simulink model "sampleModel1979_5"  (R2023a)
settings: Solver=VariableStepAuto  StartTime=0.0  StopTime=10.0  RelTol=1e-3
libraries: hdlsllib x6, simulink x2
settings Model: Creator=user1  LastModifiedBy=user1

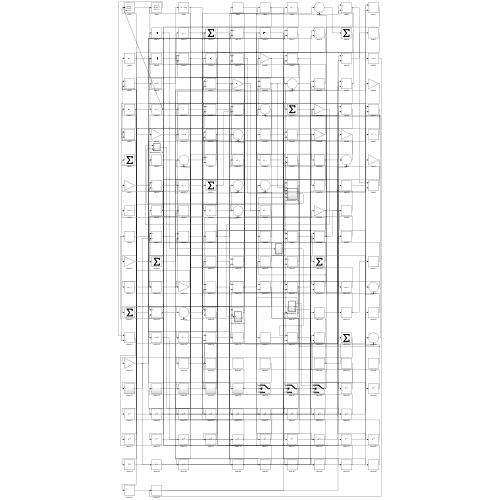
[thumbnail: Simulink's stored preview of the top-level diagram]
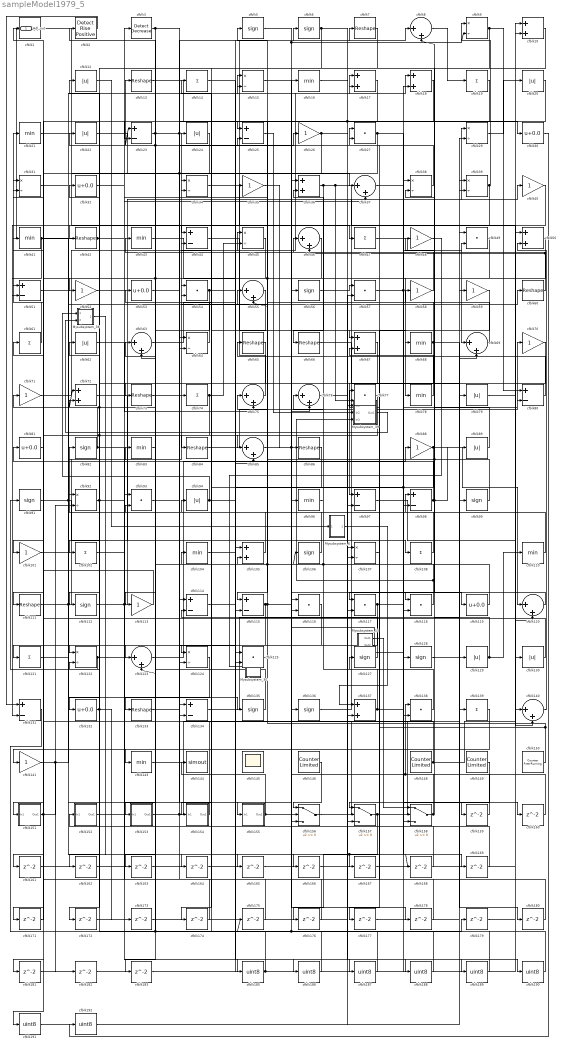
== system sampleModel1979_5 ==
  Mysubsystem_15 : Subsystem  TreatAsAtomicUnit=on  RTWFcnName=Mysubsystem_15
      settings: RTWFcnNameOpts=User specified  RTWFileNameOpts=Use function name
  Mysubsystem_30 : Subsystem  TreatAsAtomicUnit=on  RTWFcnName=Mysubsystem_30
      settings: RTWFcnNameOpts=User specified  RTWFileNameOpts=Use function name
  Mysubsystem_36 : Subsystem  TreatAsAtomicUnit=on  RTWFcnName=Mysubsystem_36
      settings: RTWFcnNameOpts=User specified  RTWFileNameOpts=Use function name
  Mysubsystem_39 : Subsystem  TreatAsAtomicUnit=on  RTWFcnName=Mysubsystem_39
      settings: RTWFcnNameOpts=User specified  RTWFileNameOpts=Use function name
  Mysubsystem_6 : Subsystem  TreatAsAtomicUnit=on  RTWFcnName=Mysubsystem_6
      settings: RTWFcnNameOpts=User specified  RTWFileNameOpts=Use function name
  cfblk1 : simulink/Logic and Bit Operations/Bit Set  iBit=0
      settings: LibrarySourceBlock=|
      | hdlsllib/Logic and Bit
      | Operations/Bit Set
  cfblk{10,17..18,36,50,67,72,105,137} (9 alike) : Sum  OutDataTypeStr=uint8
  cfblk{26,35,40,48,52,58..59,70..71,88,101,113,141} (13 alike) : Gain  OutDataTypeStr=uint8
  cfblk{14,19,47,61,74,102,108,121,139} (9 alike) : Sum  Inputs=+  OutDataTypeStr=uint8
  cfblk{16,21,41,43,68,78,83,96,104,110,143} (11 alike) : MinMax  OutDataTypeStr=uint8
  cfblk{5..6,56,82,91,99,106,112,127..128,135..136} (12 alike) : Signum
  cfblk{9,15,29,31,34,38..39,45,64,92,107,122,124} (13 alike) : Product  Inputs=*/  OutDataTypeStr=uint8  RndMeth=Zero  SaturateOnIntegerOverflow=on
  cfblk{7,13,42,60,65..66,73,84,86,111,133} (11 alike) : Reshape
  cfblk{23,25,44,51,80,97..98,114..115,131,134} (11 alike) : Sum  Inputs=+-  OutDataTypeStr=uint8
  cfblk{27,49,54,57,77,93,116..118,125,138} (11 alike) : DotProduct  OutDataTypeStr=uint8
  cfblk{30,32,53,81,119,132} (6 alike) : Bias  Bias=0.0  SaturateOnIntegerOverflow=off
  cfblk{12,20,22,24,62,79,89,94,129..130} (10 alike) : Abs  OutDataTypeStr=uint8  SaturateOnIntegerOverflow=off
  cfblk{8,37,46,55,63,69,75..76,85,120,123,140} (12 alike) : Sum  Inputs=|++  OutDataTypeStr=uint8
  cfblk144 : ToWorkspace  VariableName=simout  SaveFormat=Timeseries  SampleTime=-1
  cfblk145 : Scope
      settings: Floating=on
  cfblk146 : hdlsllib/Sources/Counter Limited  uplimit=7  tsamp=-1
  cfblk148 : hdlsllib/Sources/Counter Limited  uplimit=7  tsamp=-1
  cfblk149 : hdlsllib/Sources/Counter Limited  uplimit=7  tsamp=-1
  cfblk150 : hdlsllib/Sources/Counter Free-Running  NumBits=16  tsamp=-1
  cfblk151 : Subsystem
      settings: LibrarySourceBlock=|
      | hdlsllib/Ports &
      | Subsystems/Subsystem
  cfblk152 : Subsystem
      settings: LibrarySourceBlock=|
      | hdlsllib/Ports &
      | Subsystems/Subsystem
  cfblk153 : Subsystem
      settings: LibrarySourceBlock=|
      | hdlsllib/Ports &
      | Subsystems/Subsystem
  cfblk154 : Subsystem
      settings: LibrarySourceBlock=|
      | hdlsllib/Ports &
      | Subsystems/Subsystem
  cfblk155 : Subsystem
      settings: LibrarySourceBlock=|
      | hdlsllib/Ports &
      | Subsystems/Subsystem
  cfblk156 : Switch  OutDataTypeStr=uint8  SaturateOnIntegerOverflow=off  InputSameDT=off
  cfblk157 : Switch  OutDataTypeStr=uint8  SaturateOnIntegerOverflow=off  InputSameDT=off
  cfblk158 : Switch  OutDataTypeStr=uint8  SaturateOnIntegerOverflow=off  InputSameDT=off
  cfblk{159..169,171..183} (24 alike) : Delay  SampleTime=1
  cfblk{185..192} (8 alike) : DataTypeConversion  OutDataTypeStr=uint8  SaturateOnIntegerOverflow=off  RndMeth=Floor
  cfblk2 : hdlsllib/Logic and Bit Operations/Detect Rise Positive  vinit=0  OutDataTypeStr=uint8
  cfblk3 : simulink/Logic and Bit Operations/Detect Decrease  vinit=0.0  OutDataTypeStr=uint8
      settings: LibrarySourceBlock=|
      | hdlsllib/Logic and Bit
      | Operations/Detect
      | Decrease
  Hdl_out : Outport  OutDataTypeStr=uint8
  wires:
  cfblk35/1 -> cfblk86/1
  cfblk75/1 -> cfblk6/1
  cfblk115/1 -> cfblk55/2, cfblk76/2, cfblk121/1
  cfblk150/1 -> cfblk75/1, cfblk127/1
  cfblk38/1 -> cfblk13/1
  cfblk106/1 -> cfblk82/1
  cfblk136/1 -> cfblk29/1
  cfblk112/1 -> cfblk40/1, cfblk15/2
  cfblk94/1 -> Mysubsystem_36/1(In1), cfblk7/1
  cfblk58/1 -> cfblk43/1
  cfblk73/1 -> cfblk24/1
  cfblk61/1 -> cfblk21/1
  cfblk102/1 -> cfblk34/1
  cfblk40/1 -> cfblk42/1
  cfblk1/1 -> cfblk96/1
  cfblk3/1 -> cfblk143/1, cfblk125/2
  cfblk77/1 -> cfblk122/1, cfblk151/1(In1)
  cfblk99/1 -> cfblk54/1, cfblk58/1
  cfblk137/1 -> cfblk106/1, cfblk76/1, cfblk169/1
  cfblk47/1 -> cfblk69/1
  cfblk122/1 -> cfblk91/1, cfblk186/1
  cfblk24/1 -> cfblk113/1
  cfblk70/1 -> cfblk97/1
  cfblk120/1 -> cfblk117/1
  cfblk29/1 -> cfblk20/1
  cfblk107/1 -> cfblk77/1
  cfblk52/1 -> cfblk18/1
  cfblk53/1 -> cfblk45/1
  cfblk123/1 -> cfblk88/1
  cfblk54/1 -> cfblk98/2, cfblk163/1
  cfblk84/1 -> cfblk70/1
  cfblk45/1 -> cfblk141/1, cfblk183/1
  cfblk111/1 -> cfblk74/1, cfblk17/2
  cfblk69/1 -> cfblk34/2
  cfblk153/1(Out1) -> cfblk99/1, cfblk8/1
  cfblk158/1 -> cfblk138/1, cfblk67/2, cfblk98/1
  cfblk60/1 -> cfblk46/1, cfblk46/2
  cfblk49/1 -> cfblk78/1
  cfblk39/1 -> cfblk9/1, cfblk51/2
  cfblk74/1 -> cfblk134/2, cfblk45/2
  cfblk56/1 -> cfblk57/1
  cfblk105/1 -> cfblk92/1
  cfblk13/1 -> cfblk25/1
  cfblk19/1 -> cfblk84/1
  cfblk6/1 -> cfblk112/1, cfblk119/1
  cfblk86/1 -> cfblk154/1(In1)
  cfblk129/1 -> cfblk48/1, cfblk110/1
  cfblk27/1 -> cfblk64/2, cfblk160/1
  cfblk135/1 -> cfblk71/1
  cfblk143/1 -> cfblk38/1
  cfblk110/1 -> cfblk94/1
  cfblk156/1 -> cfblk39/1
  cfblk149/1 -> cfblk157/1
  cfblk71/1 -> cfblk16/1
  cfblk130/1 -> cfblk61/1
  cfblk7/1 -> cfblk102/1
  cfblk118/1 -> Mysubsystem_39/3(In3), cfblk63/1
  cfblk132/1 -> cfblk172/1, cfblk173/1
  cfblk141/1 -> cfblk60/1, cfblk182/1
  cfblk72/1 -> cfblk114/1
  cfblk42/1 -> cfblk47/1, Hdl_out/1
  cfblk18/1 -> cfblk111/1
  cfblk82/1 -> cfblk167/1, cfblk168/1, cfblk72/2
  cfblk32/1 -> cfblk3/1
  cfblk80/1 -> cfblk65/1
  cfblk121/1 -> cfblk83/1
  cfblk78/1 -> cfblk27/1
  cfblk66/1 -> cfblk129/1
  cfblk8/1 -> cfblk19/1
  cfblk34/1 -> cfblk137/2
  cfblk125/1 -> cfblk25/2
  cfblk98/1 -> cfblk89/1, cfblk8/2, cfblk81/1
  cfblk92/1 -> cfblk32/1, cfblk37/2
  cfblk138/1 -> cfblk114/2
  cfblk20/1 -> cfblk85/1
  cfblk68/1 -> cfblk73/1, cfblk22/1, cfblk180/1
  cfblk104/1 -> cfblk189/1
  cfblk46/1 -> cfblk115/1, cfblk181/1
  cfblk43/1 -> cfblk105/1
  cfblk23/1 -> cfblk30/1, cfblk37/1, cfblk123/2
  cfblk16/1 -> cfblk97/2
  cfblk2/1 -> cfblk131/1
  cfblk146/1 -> cfblk156/1
  cfblk155/1(Out1) -> cfblk144/1, cfblk178/1
  cfblk15/1 -> cfblk136/1
  cfblk14/1 -> cfblk187/1
  cfblk85/1 -> cfblk56/1, cfblk117/2
  cfblk62/1 -> cfblk75/2
  cfblk5/1 -> cfblk9/2, cfblk67/1
  cfblk127/1 -> cfblk105/2
  cfblk36/1 -> cfblk140/2, cfblk77/2, cfblk66/1
  cfblk117/1 -> cfblk80/2, cfblk161/1
  cfblk157/1 -> cfblk69/2, cfblk176/1
  cfblk37/1 -> cfblk138/2
  cfblk26/1 -> cfblk171/1, cfblk188/1
  cfblk89/1 -> cfblk38/2
  cfblk55/1 -> cfblk124/1
  cfblk64/1 -> cfblk53/1
  cfblk21/1 -> cfblk124/2, cfblk116/2
  cfblk17/1 -> Mysubsystem_39/1(In1), cfblk23/2
  cfblk67/1 -> cfblk132/1
  cfblk57/1 -> cfblk49/2, cfblk159/1
  cfblk154/1(Out1) -> cfblk31/1
  cfblk10/1 -> cfblk118/1
  cfblk133/1 -> cfblk156/2
  cfblk113/1 -> cfblk51/1
  cfblk134/1 -> cfblk79/1
  cfblk124/1 -> cfblk153/1(In1)
  cfblk9/1 -> cfblk44/1, cfblk80/1
  cfblk140/1 -> cfblk50/2
  cfblk83/1 -> cfblk133/1
  cfblk79/1 -> cfblk10/1
  cfblk44/1 -> cfblk68/1
  cfblk31/1 -> cfblk15/1
  cfblk119/1 -> cfblk2/1, cfblk23/1, cfblk5/1
  cfblk128/1 -> cfblk59/1
  cfblk116/1 -> cfblk123/1
  cfblk96/1 -> cfblk36/2
  cfblk151/1(Out1) -> cfblk41/1, cfblk92/2
  cfblk22/1 -> cfblk107/2
  cfblk41/1 -> cfblk155/1(In1), cfblk131/2
  cfblk108/1 -> cfblk55/1
  cfblk91/1 -> cfblk108/1, cfblk17/1
  cfblk88/1 -> cfblk158/2, cfblk174/1, cfblk120/1
  cfblk148/1 -> cfblk62/1, cfblk72/1, cfblk130/1
  cfblk50/1 -> cfblk52/1
  cfblk81/1 -> cfblk101/1
  cfblk97/1 -> cfblk120/2
  cfblk63/1 -> cfblk35/1
  cfblk51/1 -> cfblk135/1
  cfblk152/1(Out1) -> cfblk185/1
  cfblk93/1 -> cfblk26/1
  cfblk159/1 -> cfblk36/1
  cfblk160/1 -> cfblk49/1
  cfblk161/1 -> cfblk18/2
  cfblk65/1 -> cfblk162/1
  cfblk162/1 -> cfblk134/1
  cfblk163/1 -> cfblk29/2
  cfblk101/1 -> cfblk164/1
  cfblk164/1 -> cfblk54/2
  cfblk165/1 -> cfblk57/2
  cfblk114/1 -> cfblk166/1
  cfblk166/1 -> cfblk107/1
  cfblk167/1 -> cfblk50/1
  cfblk168/1 -> cfblk122/2
  cfblk169/1 -> cfblk44/2
  cfblk171/1 -> cfblk1/1
  cfblk172/1 -> cfblk157/2
  cfblk173/1 -> cfblk115/2
  cfblk174/1 -> cfblk64/1
  cfblk175/1 -> cfblk93/1
  cfblk176/1 -> cfblk63/2
  cfblk59/1 -> cfblk177/1
  cfblk177/1 -> cfblk39/2
  cfblk178/1 -> cfblk31/2
  cfblk131/1 -> cfblk179/1
  cfblk179/1 -> cfblk140/1
  cfblk180/1 -> cfblk27/2
  cfblk181/1 -> cfblk118/2
  cfblk182/1 -> cfblk85/2
  cfblk183/1 -> cfblk10/2
  cfblk185/1 -> cfblk125/1, cfblk128/1
  cfblk186/1 -> cfblk152/1(In1)
  cfblk187/1 -> cfblk175/1, cfblk116/1
  cfblk188/1 -> cfblk14/1
  cfblk189/1 -> cfblk93/2, cfblk12/1
  cfblk76/1 -> cfblk190/1
  cfblk190/1 -> cfblk104/1
  cfblk139/1 -> cfblk191/1
  cfblk191/1 -> cfblk157/3
  cfblk30/1 -> cfblk192/1
  cfblk192/1 -> cfblk139/1
  cfblk12/1 -> Mysubsystem_6/1(In1)
  Mysubsystem_6/1(Out1) -> cfblk137/1
  Mysubsystem_15/1(Out1) -> cfblk158/1
  Mysubsystem_15/2(Out2) -> cfblk156/3
  Mysubsystem_15/3(Out3) -> cfblk158/3
  cfblk48/1 -> Mysubsystem_30/1(U)
  Mysubsystem_36/1(Out1) -> cfblk165/1
  cfblk25/1 -> Mysubsystem_39/2(In2)
  Mysubsystem_39/1(Out1) -> Mysubsystem_36/2(In2)

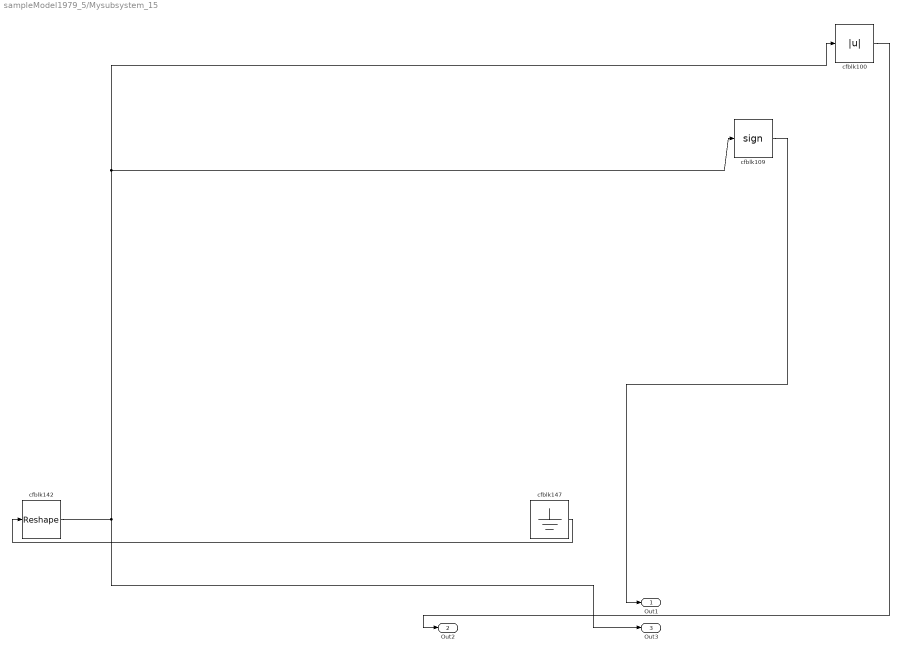
== system sampleModel1979_5/Mysubsystem_15 ==
  cfblk100 : Abs  SaturateOnIntegerOverflow=off
  cfblk109 : Signum
  cfblk142 : Reshape
  cfblk147 : Ground
  Out1 : Outport
  Out2 : Outport  Port=2
  Out3 : Outport  Port=3
  wires:
  cfblk109/1 -> Out1/1
  cfblk147/1 -> cfblk142/1
  cfblk142/1 -> Out3/1, cfblk109/1, cfblk100/1
  cfblk100/1 -> Out2/1

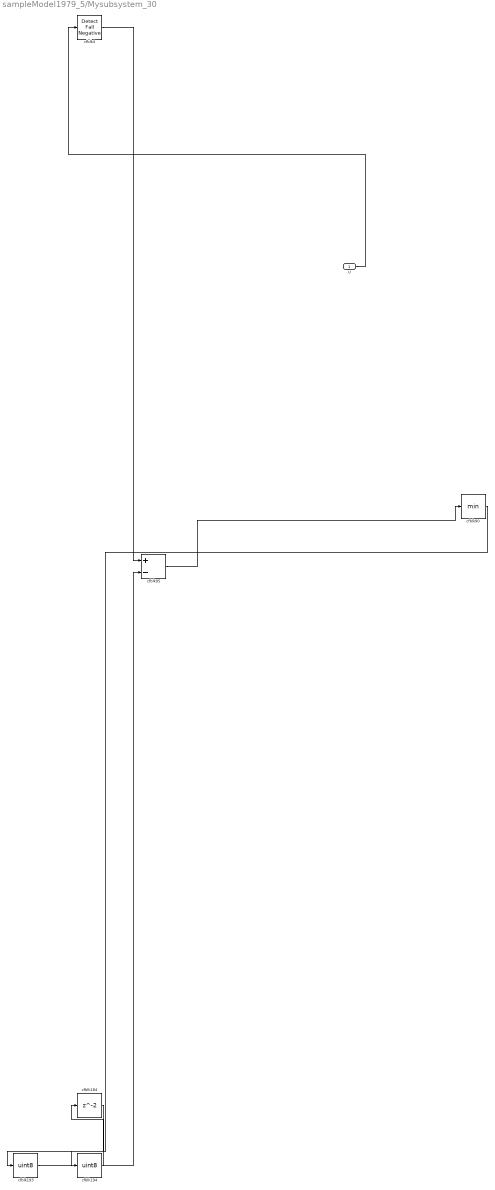
== system sampleModel1979_5/Mysubsystem_30 ==
  U : Inport
  cfblk184 : Delay  SampleTime=1
  cfblk193 : DataTypeConversion  OutDataTypeStr=uint8  SaturateOnIntegerOverflow=off  RndMeth=Floor
  cfblk194 : DataTypeConversion  OutDataTypeStr=uint8  SaturateOnIntegerOverflow=off  RndMeth=Floor
  cfblk4 : hdlsllib/Logic and Bit Operations/Detect Fall Negative  vinit=0  OutDataTypeStr=boolean
  cfblk90 : MinMax
  cfblk95 : Sum  Inputs=+-
  wires:
  cfblk184/1 -> cfblk193/1
  cfblk95/1 -> cfblk90/1
  cfblk4/1 -> cfblk95/1
  cfblk193/1 -> cfblk95/2
  cfblk194/1 -> cfblk184/1
  U/1 -> cfblk4/1
  cfblk90/1 -> cfblk194/1

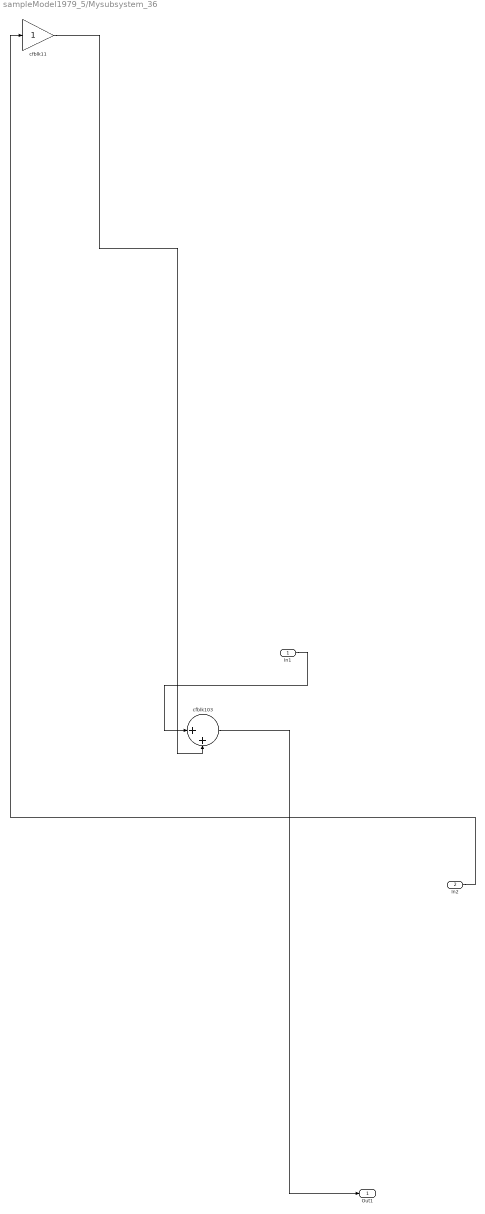
== system sampleModel1979_5/Mysubsystem_36 ==
  In1 : Inport
  In2 : Inport  Port=2
  cfblk103 : Sum  Inputs=|++
  cfblk11 : Gain
  Out1 : Outport
  wires:
  cfblk11/1 -> cfblk103/2
  In2/1 -> cfblk11/1
  In1/1 -> cfblk103/1
  cfblk103/1 -> Out1/1

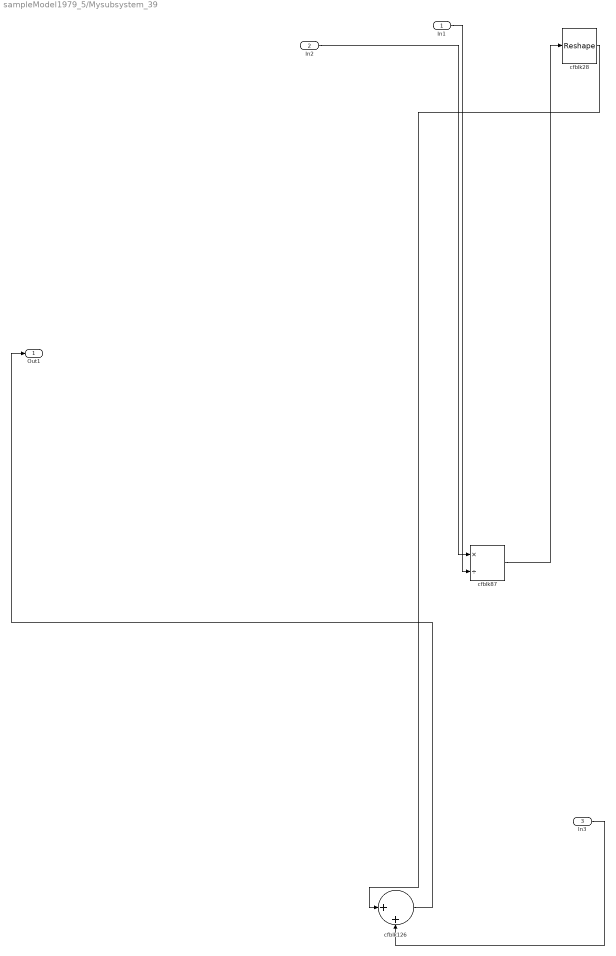
== system sampleModel1979_5/Mysubsystem_39 ==
  In1 : Inport
  In2 : Inport  Port=2
  In3 : Inport  Port=3
  cfblk126 : Sum  Inputs=|++
  cfblk28 : Reshape
  cfblk87 : Product  Inputs=*/  RndMeth=Zero  SaturateOnIntegerOverflow=on
  Out1 : Outport
  wires:
  cfblk28/1 -> cfblk126/1
  cfblk87/1 -> cfblk28/1
  In1/1 -> cfblk87/2
  cfblk126/1 -> Out1/1
  In3/1 -> cfblk126/2
  In2/1 -> cfblk87/1

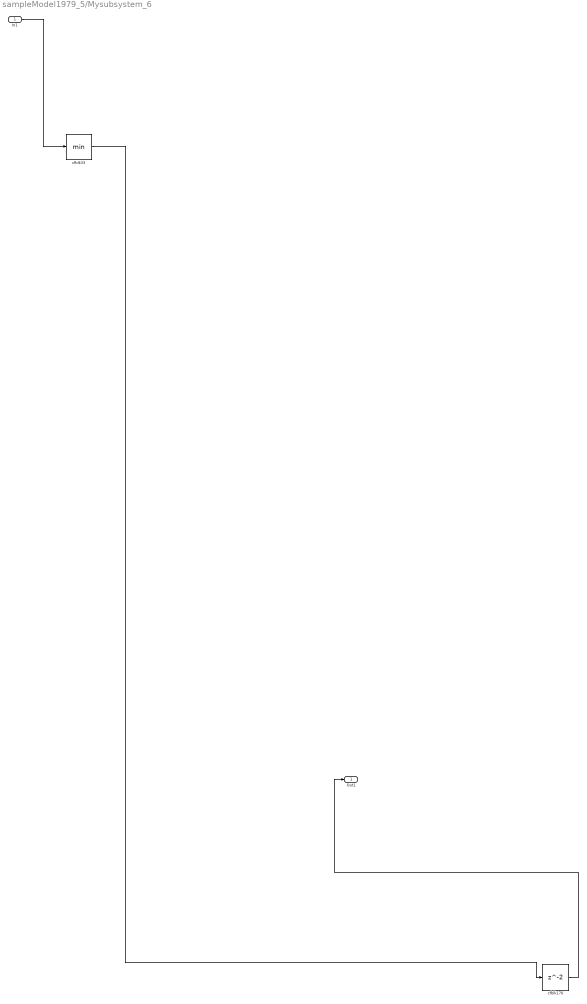
== system sampleModel1979_5/Mysubsystem_6 ==
  In1 : Inport
  cfblk170 : Delay  SampleTime=1
  cfblk33 : MinMax
  Out1 : Outport
  wires:
  cfblk33/1 -> cfblk170/1
  In1/1 -> cfblk33/1
  cfblk170/1 -> Out1/1

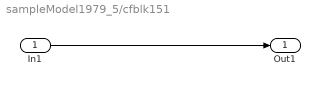
== system sampleModel1979_5/cfblk151 ==
  In1 : Inport
  Out1 : Outport
  wires:
  In1/1 -> Out1/1

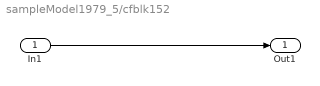
== system sampleModel1979_5/cfblk152 ==
  In1 : Inport
  Out1 : Outport
  wires:
  In1/1 -> Out1/1

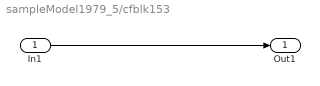
== system sampleModel1979_5/cfblk153 ==
  In1 : Inport
  Out1 : Outport
  wires:
  In1/1 -> Out1/1

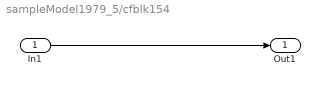
== system sampleModel1979_5/cfblk154 ==
  In1 : Inport
  Out1 : Outport
  wires:
  In1/1 -> Out1/1

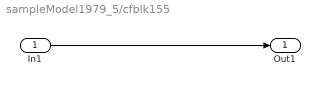
== system sampleModel1979_5/cfblk155 ==
  In1 : Inport
  Out1 : Outport
  wires:
  In1/1 -> Out1/1
